simulink model "example_mass_spring_damper_system"  (R2021a)
settings: Solver=VariableStepAuto  StartTime=0.0  StopTime=10  RelTol=1e-3
values from neighbouring files (symbols this model uses):
  b = 10    [mass_spring_damper_system.m]
  k = 400    [mass_spring_damper_system.m]
  m = massvalue(i)    [mass_spring_damper_system.m]
  x0 = 1    [mass_spring_damper_system.m]
settings Model: Creator=YasserNet  LastModifiedBy=YasserNet

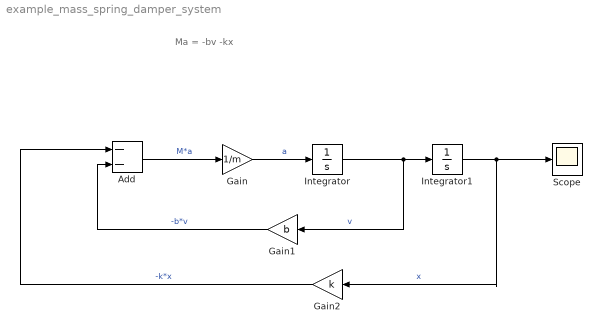
== system example_mass_spring_damper_system ==
  note: Ma = -bv -kx
  Add : Sum  Inputs=--
  Gain : Gain  Gain=1/m
  Gain1 : Gain  Gain=b
  Gain2 : Gain  Gain=k
  Integrator : Integrator
  Integrator1 : Integrator  InitialCondition=x0
  Scope : Scope
  wires:
  Add/1 -> Gain/1  "M*a"
  Gain/1 -> Integrator/1  "a"
  Integrator/1 -> Gain1/1, Integrator1/1  "v"
  Integrator1/1 -> Gain2/1, Scope/1  "x"
  Gain1/1 -> Add/2  "-b*v"
  Gain2/1 -> Add/1  "-k*x"
